simulink model "Simple_Pendulum_Motion_Simulation"  (R2024b)
settings: Solver=VariableStepAuto  StartTime=0.0  StopTime=10.0  MaxStep=1e-3  RelTol=1e-3
settings Model: Creator=Ahmad  LastModifiedBy=Ahmad

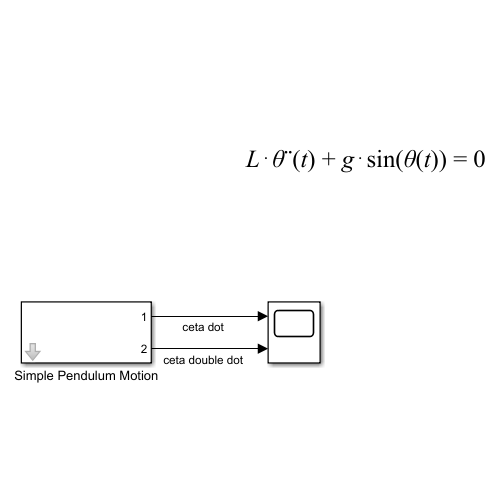
[thumbnail: Simulink's stored preview of the top-level diagram]
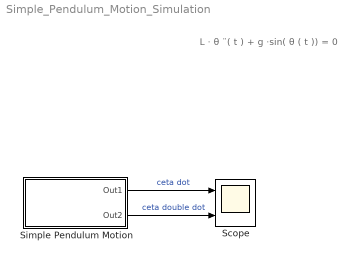
== system Simple_Pendulum_Motion_Simulation ==
  note: L ⋅ θ ¨( t ) + g ⋅sin( θ ( t )) = 0
  Scope : Scope  NumInputPorts=2
  Simple Pendulum Motion : Subsystem  mask{L=1, g=9.81}
      mask prompts: L "length"; g "Gravity"
      mask DialogControl parameter Prompt: parameters
  wires:
  Simple Pendulum Motion/1(Out1) -> Scope/1  "ceta dot"
  Simple Pendulum Motion/2(Out2) -> Scope/2  "ceta double dot"

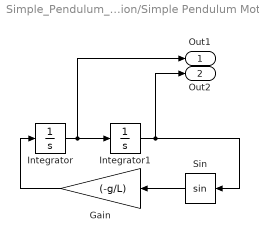
== system Simple_Pendulum_Motion_Simulation/Simple Pendulum Motion ==
  Gain : Gain  Gain=(-g/L)
  Integrator : Integrator
  Integrator1 : Integrator  InitialCondition=1
  Sin : Trigonometry
  Out1 : Outport
  Out2 : Outport  Port=2
  wires:
  Sin/1 -> Gain/1
  Integrator/1 -> Out1/1, Integrator1/1
  Integrator1/1 -> Out2/1, Sin/1
  Gain/1 -> Integrator/1
